simulink model "LyapunovControl"  (R2015a)
settings: Solver=ode5  StartTime=0.0  StopTime=15  FixedStep=0.001  RelTol=1e-3
values from neighbouring files (symbols this model uses):
  Kt = 10    [Init.m]
  Kx = 10    [Init.m]
  Ky = 15    [Init.m]
  L = 0.13    [Init.m]    (also in KinematicPlot.m; plotVehicle.m)
  L_e = (1 + err_L)*L    (= 0.13)    [Init.m]
  r = 0.1    [Init.m]    (also in KinematicPlot.m)
  R = 2    [Init.m]
  r_e = (1 + err_r)*r    (= 0.1)    [Init.m]
  theta0 = pi    (= 3.14159265359)    [Init.m]
  wd = 0.5    [Init.m]
  x0 = 2.3    [Init.m]
  y0 = 0    [Init.m]
undefined symbols (not defined in the file): d
settings Model: Creator=tgvo  LastModifiedBy=tgvo
settings DataIOCC: LimitDataPoints=off

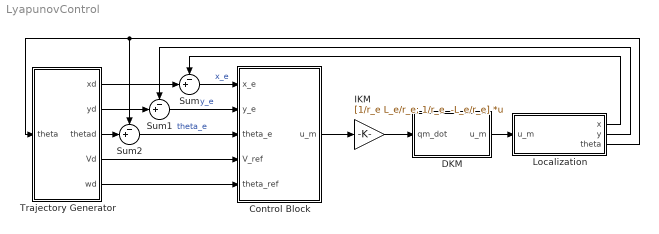
== system LyapunovControl ==
  Control Block : Subsystem  mask{Kx=Kx, Ky=Ky, Kt=Kt}
      mask prompts: Kt "Ktheta"
  DKM : Subsystem  mask{r=r, L=L}
      mask prompts: r "Wheel Raidus (r)"; L "Half of Track Gauge (L)"
  IKM : Gain  Gain="[1/r_e L_e/r_e; 1/r_e  -L_e/r_e]"  Multiplication=Matrix(K*u) (u vector)
  Localization : Subsystem  mask{x0=x0, y0=y0, theta0=theta0, d=d}
      mask prompts: x0 "Initial value of x (x0)"; y0 "Initial value of y (y0)"; theta0 "Initial value of theta (theta0)"; d "Distqnce b/w P and Om"
  Sum : Sum  Inputs=-+|
  Sum1 : Sum  Inputs=-+|
  Sum2 : Sum  Inputs=-+|
  Trajectory Generator : Subsystem  mask{R=R, wd=wd}
      mask prompts: R "Trajectory Radius (R)"; wd "Desired Angular Velocity (wd)"
  wires:
  Trajectory Generator/1(xd) -> Sum/2
  Trajectory Generator/2(yd) -> Sum1/2
  Sum/1 -> Control Block/1(x_e)  "x_e"
  Sum1/1 -> Control Block/2(y_e)  "y_e"
  Sum2/1 -> Control Block/3(theta_e)  "theta_e"
  Trajectory Generator/4(Vd) -> Control Block/4(V_ref)
  Trajectory Generator/5(wd) -> Control Block/5(theta_ref)
  Control Block/1(u_m) -> IKM/1
  IKM/1 -> DKM/1(qm_dot)
  DKM/1("u_m ") -> Localization/1(u_m)
  Localization/3(theta) -> Trajectory Generator/1(theta), Sum2/1
  Localization/1(x) -> Sum/1
  Localization/2(y) -> Sum1/1
  Trajectory Generator/3(thetad) -> Sum2/2

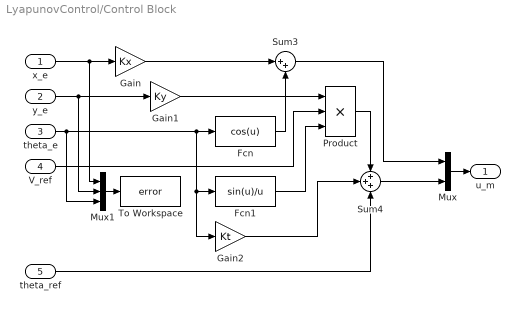
== system LyapunovControl/Control Block ==
  x_e : Inport
  y_e : Inport  Port=2
  theta_e : Inport  Port=3
  V_ref : Inport  Port=4
  theta_ref : Inport  Port=5
  Fcn : Fcn  Expr=cos(u)
  Fcn1 : Fcn  Expr=sin(u)/u
  Gain : Gain  Gain=Kx
  Gain1 : Gain  Gain=Ky
  Gain2 : Gain  Gain=Kt
  Mux : Mux  Inputs=2
  Mux1 : Mux  Inputs=3
  Product : Product  Inputs=3
  Sum3 : Sum  Inputs=|++
  Sum4 : Sum  Inputs=+++
  To Workspace : ToWorkspace  VariableName=error  SampleTime=-1
  u_m : Outport
  wires:
  V_ref/1 -> Product/2
  Sum4/1 -> Mux/2
  Fcn/1 -> Sum3/2
  Gain/1 -> Sum3/1
  Sum3/1 -> Mux/1
  Product/1 -> Sum4/1
  Gain2/1 -> Sum4/2
  Mux/1 -> u_m/1
  Gain1/1 -> Product/1
  theta_ref/1 -> Sum4/3
  Fcn1/1 -> Product/3
  x_e/1 -> Mux1/1, Gain/1
  y_e/1 -> Gain1/1, Mux1/2
  theta_e/1 -> Gain2/1, Fcn1/1, Fcn/1, Mux1/3
  Mux1/1 -> To Workspace/1

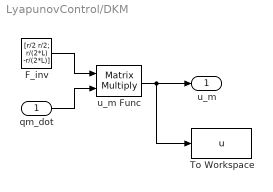
== system LyapunovControl/DKM ==
  qm_dot : Inport
  F_inv : Constant  Value=[r/2 r/2; r/(2*L) -r/(2*L)]
  To Workspace : ToWorkspace  VariableName=u  SampleTime=-1
  u_m Func : Product  Multiplication=Matrix(*)
  "u_m " : Outport
  wires:
  F_inv/1 -> u_m Func/1
  u_m Func/1 -> To Workspace/1, "u_m "/1
  qm_dot/1 -> u_m Func/2

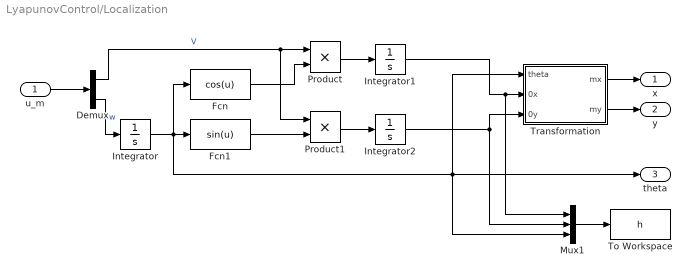
== system LyapunovControl/Localization ==
  u_m : Inport
  Demux : Demux  Outputs=2
  Fcn : Fcn  Expr=cos(u)
  Fcn1 : Fcn  Expr=sin(u)
  Integrator : Integrator  InitialCondition=theta0
  Integrator1 : Integrator  InitialCondition=x0
  Integrator2 : Integrator  InitialCondition=y0
  Mux1 : Mux  Inputs=3
  Product : Product
  Product1 : Product
  To Workspace : ToWorkspace  VariableName=h  SampleTime=-1
  Transformation : Subsystem
  x : Outport
  y : Outport  Port=2
  theta : Outport  Port=3
  wires:
  Demux/2 -> Integrator/1  "w"
  u_m/1 -> Demux/1
  Fcn/1 -> Product/2
  Fcn1/1 -> Product1/2
  Integrator/1 -> Mux1/3, Transformation/1(theta), theta/1, Fcn/1, Fcn1/1
  Demux/1 -> Product1/1, Product/1  "V"
  Product/1 -> Integrator1/1
  Product1/1 -> Integrator2/1
  Integrator1/1 -> Mux1/1, Transformation/2(0x)
  Integrator2/1 -> Transformation/3(0y), Mux1/2
  Transformation/1(mx) -> x/1
  Transformation/2(my) -> y/1
  Mux1/1 -> To Workspace/1

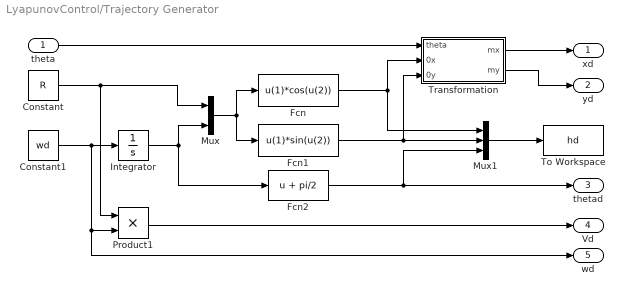
== system LyapunovControl/Trajectory Generator ==
  theta : Inport
  Constant : Constant  Value=R
  Constant1 : Constant  Value=wd
  Fcn : Fcn  Expr=u(1)*cos(u(2))
  Fcn1 : Fcn  Expr=u(1)*sin(u(2))
  Fcn2 : Fcn  Expr=u + pi/2
  Integrator : Integrator
  Mux : Mux  Inputs=2
  Mux1 : Mux  Inputs=3
  Product1 : Product
  To Workspace : ToWorkspace  VariableName=hd  SampleTime=-1
  Transformation : Subsystem
  xd : Outport
  yd : Outport  Port=2
  thetad : Outport  Port=3
  Vd : Outport  Port=4
  wd : Outport  Port=5
  wires:
  Product1/1 -> Vd/1
  Integrator/1 -> Fcn2/1, Mux/2
  Constant/1 -> Product1/1, Mux/1
  Constant1/1 -> Integrator/1, wd/1, Product1/2
  Mux/1 -> Fcn/1, Fcn1/1
  Fcn/1 -> Mux1/1, Transformation/2(0x)
  Fcn1/1 -> Transformation/3(0y), Mux1/2
  Transformation/2(my) -> yd/1
  Transformation/1(mx) -> xd/1
  theta/1 -> Transformation/1(theta)
  Mux1/1 -> To Workspace/1
  Fcn2/1 -> thetad/1, Mux1/3

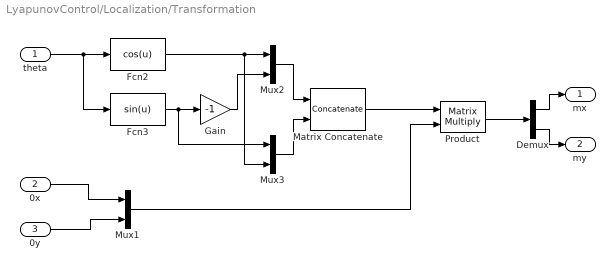
== system LyapunovControl/Localization/Transformation ==
  theta : Inport
  0x : Inport  Port=2
  0y : Inport  Port=3
  Demux : Demux  Outputs=2
  Fcn2 : Fcn  Expr=cos(u)
  Fcn3 : Fcn  Expr=sin(u)
  Gain : Gain  Gain=-1
  Matrix Concatenate : Concatenate  Mode=Multidimensional array  ConcatenateDimension=2
  Mux1 : Mux  Inputs=2
  Mux2 : Mux  Inputs=2
  Mux3 : Mux  Inputs=2
  Product : Product  Multiplication=Matrix(*)
  mx : Outport
  my : Outport  Port=2
  wires:
  Fcn3/1 -> Mux3/1, Gain/1
  Mux3/1 -> Matrix Concatenate/2
  Mux2/1 -> Matrix Concatenate/1
  theta/1 -> Fcn3/1, Fcn2/1
  Gain/1 -> Mux2/2
  Matrix Concatenate/1 -> Product/1
  Fcn2/1 -> Mux3/2, Mux2/1
  0x/1 -> Mux1/1
  0y/1 -> Mux1/2
  Mux1/1 -> Product/2
  Demux/1 -> mx/1
  Demux/2 -> my/1
  Product/1 -> Demux/1

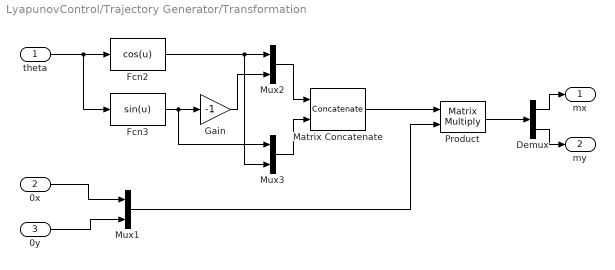
== system LyapunovControl/Trajectory Generator/Transformation ==
  theta : Inport
  0x : Inport  Port=2
  0y : Inport  Port=3
  Demux : Demux  Outputs=2
  Fcn2 : Fcn  Expr=cos(u)
  Fcn3 : Fcn  Expr=sin(u)
  Gain : Gain  Gain=-1
  Matrix Concatenate : Concatenate  Mode=Multidimensional array  ConcatenateDimension=2
  Mux1 : Mux  Inputs=2
  Mux2 : Mux  Inputs=2
  Mux3 : Mux  Inputs=2
  Product : Product  Multiplication=Matrix(*)
  mx : Outport
  my : Outport  Port=2
  wires:
  Fcn3/1 -> Mux3/1, Gain/1
  Mux3/1 -> Matrix Concatenate/2
  Mux2/1 -> Matrix Concatenate/1
  theta/1 -> Fcn3/1, Fcn2/1
  Gain/1 -> Mux2/2
  Matrix Concatenate/1 -> Product/1
  Fcn2/1 -> Mux3/2, Mux2/1
  0x/1 -> Mux1/1
  0y/1 -> Mux1/2
  Mux1/1 -> Product/2
  Demux/1 -> mx/1
  Demux/2 -> my/1
  Product/1 -> Demux/1
